simulink model "TS02_start"  (R2022b)
settings: Solver=ode45  StartTime=0.0  StopTime=3*60  RelTol=1e-3  EnableMultiTasking=on
undefined symbols (not defined in the file): Advantech, PCI
libraries: sldrtlib x4
settings Model: Creator=Admin  LastModifiedBy=MT
settings SolverCC: AlgebraicLoopSolver=TrustRegion
settings DataIOCC: LimitDataPoints=on  SaveFormat=Array  ReturnWorkspaceOutputs=off
settings OptimizationCC: LifeSpan=inf
settings DebuggingCC: UnconnectedInputMsg=warning  UnconnectedOutputMsg=warning  UnconnectedLineMsg=warning  SFUnexpectedBacktrackingDiag=warning  SFNoUnconditionalDefaultTransitionDiag=warning  SFExecutionAtInitializationDiag=none  SFMachineParentedDataDiag=warning  ArithmeticOperatorsInVariantConditions=warning
settings HardwareCC: ProdBitPerPointer=32  ProdBitPerSizeT=32  ProdBitPerPtrDiffT=32  ProdLargestAtomicFloat=None  ProdIntDivRoundTo=Undefined  ProdEndianess=Unspecified  ProdWordSize=32  ProdHWDeviceType=32-bit Generic
settings ModelReferenceCC: PropagateSignalLabelsOutOfModel=off
settings SFSimCC: SimUseLocalCustomCode=off  CustomCodeUndefinedFunction=UseInterfaceOnly
settings RTWCC: RTWUseLocalCustomCode=off
settings CodeAppCC: StateflowObjectComments=on
settings GRTTargetCC: TargetLangStandard=C89/C90 (ANSI)
settings ConfigComp: CovMetricSettings=dw  CovSaveCumulativeToWorkspaceVar=on  CovSaveSingleToWorkspaceVar=on  CovExternalEMLEnable=off

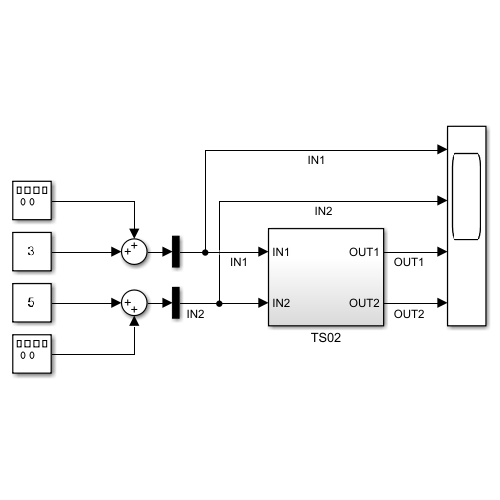
[thumbnail: Simulink's stored preview of the top-level diagram]
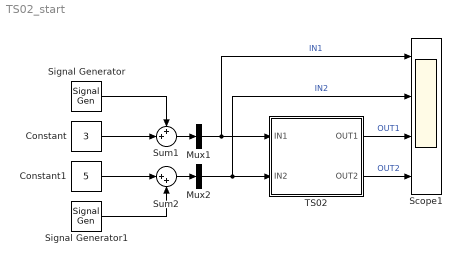
== system TS02_start ==
  Constant : Constant  Value=3
  Constant1 : Constant  Value=5
  Mux1 : Mux  Inputs=1
  Mux2 : Mux  Inputs=1
  Scope1 : Scope  NumInputPorts=4
  Signal Generator : SignalGenerator  WaveForm=square  Frequency=1/10
  Signal Generator1 : SignalGenerator  Frequency=1/10
  Sum1 : Sum  Inputs=++|
  Sum2 : Sum  Inputs=|++
  TS02 : Subsystem
  wires:
  Mux2/1 -> Scope1/2, TS02/2(IN2)  "IN2"
  Mux1/1 -> Scope1/1, TS02/1(IN1)  "IN1"
  TS02/2(OUT2) -> Scope1/4  "OUT2"
  TS02/1(OUT1) -> Scope1/3  "OUT1"
  Sum1/1 -> Mux1/1
  Sum2/1 -> Mux2/1
  Constant1/1 -> Sum2/1
  Constant/1 -> Sum1/2
  Signal Generator/1 -> Sum1/1
  Signal Generator1/1 -> Sum2/2

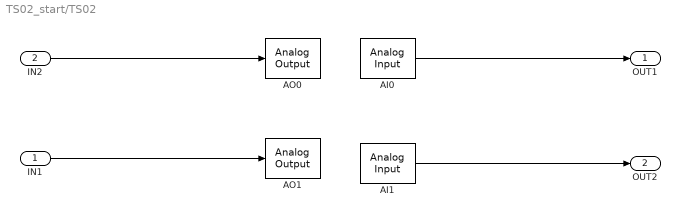
== system TS02_start/TS02 ==
  IN1 : Inport
  IN2 : Inport  Port=2
  AI0 : sldrtlib/Analog Input  SampleTime=0.1  MaxMissedTicks=10  ShowMissedTicks=off  YieldWhenWaiting=off  DrvName=Advantech/PCI-1711  DrvAddress=4294967295  DrvOptions=zeros(1,0)  Channels=1  RangeMode=1  VoltRange=1  DataType=1
      settings: AttributesFormatString=Advantech\nPCI-1711 [auto]
  AI1 : sldrtlib/Analog Input  SampleTime=0.1  MaxMissedTicks=10  ShowMissedTicks=off  YieldWhenWaiting=off  DrvName=Advantech/PCI-1711  DrvAddress=4294967295  DrvOptions=zeros(1,0)  Channels=2  RangeMode=1  VoltRange=1  DataType=1
      settings: AttributesFormatString=Advantech\nPCI-1711 [auto]
  AO0 : sldrtlib/Analog Output  SampleTime=0.1  MaxMissedTicks=10  ShowMissedTicks=off  YieldWhenWaiting=off  DrvName=Advantech/PCI-1711  DrvAddress=4294967295  DrvOptions=zeros(1,0)  Channels=1  RangeMode=1  VoltRange=2  InitialValue=[]  FinalValue=[]
      settings: AttributesFormatString=Advantech\nPCI-1711 [auto]
  AO1 : sldrtlib/Analog Output  SampleTime=0.1  MaxMissedTicks=10  ShowMissedTicks=off  YieldWhenWaiting=off  DrvName=Advantech/PCI-1711  DrvAddress=4294967295  DrvOptions=zeros(1,0)  Channels=2  RangeMode=1  VoltRange=2  InitialValue=[]  FinalValue=[]
      settings: AttributesFormatString=Advantech\nPCI-1711 [auto]
  OUT1 : Outport
  OUT2 : Outport  Port=2
  wires:
  IN2/1 -> AO0/1
  IN1/1 -> AO1/1
  AI0/1 -> OUT1/1
  AI1/1 -> OUT2/1
